simulink model "sistema2"  (R2026a)
settings: Solver=VariableStepAuto  StopTime=10
libraries: simulink x1, slpidlib x1

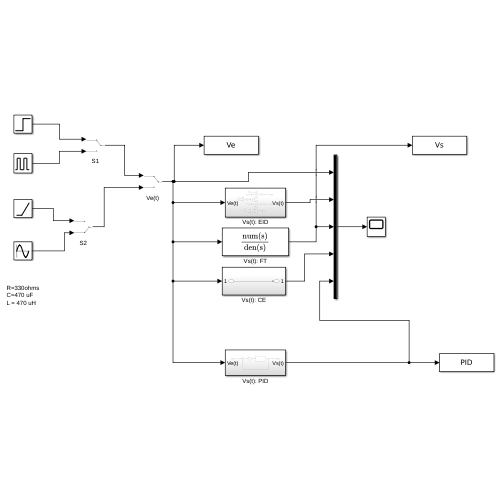
[thumbnail: Simulink's stored preview of the top-level diagram]
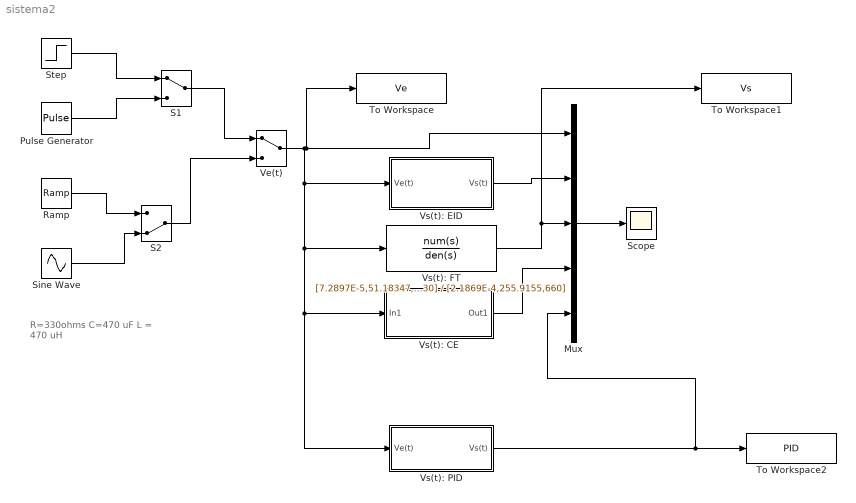
== system sistema2 ==
  note: R=330ohms
      | C=470 uF
      | L = 470 uH
  Mux : Mux  Inputs=5
  Pulse Generator : DiscretePulseGenerator  PulseType=Time based  Period=10  PulseWidth=10  PhaseDelay=1
  Ramp : simulink/Sources/Ramp  slope=1/10  start=0  InitialOutput=0
  S1 : ManualSwitch
  S2 : ManualSwitch  CurrentSetting=0
  Scope : Scope
      settings: ActiveDisplayYMinimum=-1.104134739416077  ActiveDisplayYMaximum=2.0672934495653212
  Sine Wave : Sin  Frequency=pi/2  SampleTime=0
  Step : Step  Time=0  SampleTime=0
  To Workspace : ToWorkspace  VariableName=Ve  SampleTime=-1
  To Workspace1 : ToWorkspace  VariableName=Vs  SampleTime=-1
  To Workspace2 : ToWorkspace  VariableName=PID  SampleTime=-1
  Ve(t) : ManualSwitch
  Vs(t): CE : Subsystem
  Vs(t): EID : Subsystem
  Vs(t): FT : TransferFcn  Numerator=[7.2897E-5,51.18347,330]  Denominator=[2.1869E-4,255.9155,660]
  Vs(t): PID : Subsystem
  wires:
  Vs(t): PID/1(Vs(t)) -> To Workspace2/1, Mux/5
  Mux/1 -> Scope/1
  S2/1 -> Ve(t)/2
  Ramp/1 -> S2/1
  Pulse Generator/1 -> S1/2
  Vs(t): CE/1(Out1) -> Mux/4
  Step/1 -> S1/1
  Vs(t): FT/1 -> To Workspace1/1, Mux/3
  S1/1 -> Ve(t)/1
  Vs(t): EID/1(Vs(t)) -> Mux/2
  Sine Wave/1 -> S2/2
  Ve(t)/1 -> Vs(t): EID/1(Ve(t)), Vs(t): FT/1, Vs(t): PID/1(Ve(t)), Vs(t): CE/1(In1), To Workspace/1, Mux/1

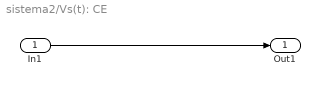
== system sistema2/Vs(t): CE ==
  In1 : Inport
  Out1 : Outport
  wires:
  In1/1 -> Out1/1

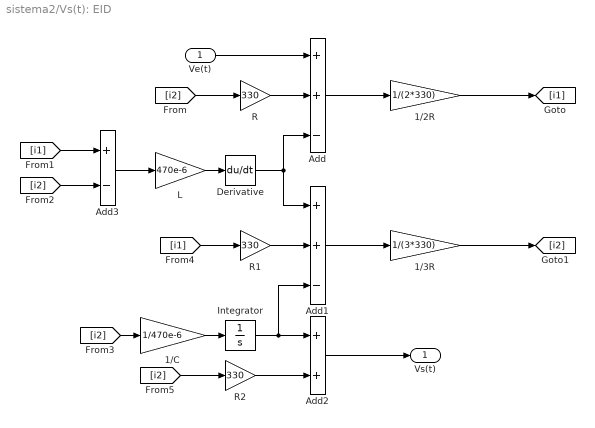
== system sistema2/Vs(t): EID ==
  Ve(t) : Inport
  1/2R : Gain  Gain=1/(2*330)
  1/3R : Gain  Gain=1/(3*330)
  1/C : Gain  Gain=1/470e-6
  Add : Sum  Inputs=++-
  Add1 : Sum  Inputs=++-
  Add2 : Sum
  Add3 : Sum  Inputs=+-
  Derivative : Derivative
  Integrator : Integrator
  L : Gain  Gain=470e-6
  R : Gain  Gain=330
  R1 : Gain  Gain=330
  R2 : Gain  Gain=330
  Vs(t) : Outport
  wires:
  Ve(t)/1 -> Add/1
  Add1/1 -> 1/3R/1
  1/3R/1 -> [i2]
  Add/1 -> 1/2R/1
  1/2R/1 -> [i1]
  R/1 -> Add/2
  [i2] -> R/1
  Derivative/1 -> Add1/1, Add/3
  R1/1 -> Add1/2
  Add3/1 -> L/1
  L/1 -> Derivative/1
  [i2] -> Add3/2
  [i1] -> Add3/1
  Integrator/1 -> Add1/3, Add2/1
  [i2] -> 1/C/1
  1/C/1 -> Integrator/1
  [i1] -> R1/1
  [i2] -> R2/1
  R2/1 -> Add2/2
  Add2/1 -> Vs(t)/1

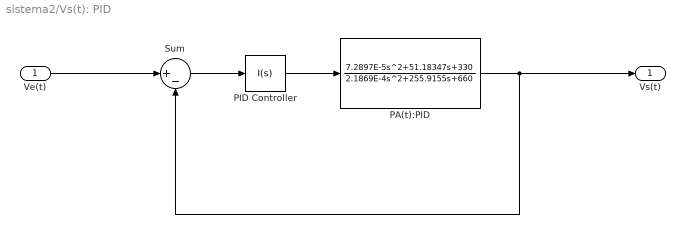
== system sistema2/Vs(t): PID ==
  Ve(t) : Inport
  PA(t):PID : TransferFcn  Numerator=[7.2897E-5,51.18347,330]  Denominator=[2.1869E-4,255.9155,660]
  PID Controller : slpidlib/PID Controller  Controller=I  Form=Parallel  TimeDomain=Continuous-time  UseExternalTs=off  SampleTime=-1  IntegratorMethod=Forward Euler  FilterMethod=Forward Euler  ControllerParametersSource=internal  P=289.6613  I=608.5886  UseKiTs=off  D=0.39134  UseExternalDerivativeSource=off  N=502.9743  UseFilter=on  TunerSelectOption=Transfer Function Based (PID Tuner App)  InitialConditionSource=internal  InitialConditionForIntegrator=0  InitialConditionForFilter=0  DifferentiatorICPrevScaledInput=0  ExternalReset=none  TrackingMode=off  Kt=1  LimitOutput=off  SatLimitsSource=internal  UpperSaturationLimit=inf  LowerSaturationLimit=-inf  LinearizeAsGain=on  AntiWindupMode=none  Kb=1  LimitIntegrator=off  UpperIntegratorSaturationLimit=inf  LowerIntegratorSaturationLimit=-inf  POutMin=[]  POutMax=[]  IOutMin=[]  IOutMax=[]  DOutMin=[]  DOutMax=[]  NOutMin=[]  NOutMax=[]  SumOutMin=[]  SumOutMax=[]  SaturationOutMin=[]  SaturationOutMax=[]  PParamMin=[]  PParamMax=[]  IParamMin=[]  IParamMax=[]  DParamMin=[]  DParamMax=[]  NParamMin=[]  NParamMax=[]  KbParamMin=[]  KbParamMax=[]  KtParamMin=[]  KtParamMax=[]  KbOutMin=[]  KbOutMax=[]  KtOutMin=[]  KtOutMax=[]  IntegratorOutMin=[]  IntegratorOutMax=[]  FilterOutMin=[]  FilterOutMax=[]  SumI1OutMin=[]  SumI1OutMax=[]  SumI2OutMin=[]  SumI2OutMax=[]  SumI3OutMin=[]  SumI3OutMax=[]  SumI4OutMin=[]  SumI4OutMax=[]  SumDOutMin=[]  SumDOutMax=[]  DifferentiatorOutMin=[]  DifferentiatorOutMax=[]  FilterDiffOutCoefMin=[]  FilterDiffOutCoefMax=[]  ReciprocalOutMin=[]  ReciprocalOutMax=[]  SumDenOutMin=[]  SumDenOutMax=[]  SumNumOutMin=[]  SumNumOutMax=[]  DivideOutMin=[]  DivideOutMax=[]  UdiffTsProdOutMin=[]  UdiffTsProdOutMax=[]  NTsProdOutMin=[]  NTsProdOutMax=[]  UintegralTsProdOutMin=[]  UintegralTsProdOutMax=[]  UngainTsProdOutMin=[]  UngainTsProdOutMax=[]  ClampingZeroOutDataTypeStr=Inherit: Inherit via back propagation  ClampingZeroOutMin=[]  ClampingZeroOutMax=[]  FilterDenConstantOutDataTypeStr=Inherit: Inherit via back propagation  FilterDenConstantOutMin=[]  FilterDenConstantOutMax=[]  PCopyOutDataTypeStr=Inherit: Inherit via back propagation  PCopyOutMin=[]  PCopyOutMax=[]  NCopyOutDataTypeStr=Inherit: Inherit via back propagation  NCopyOutMin=[]  NCopyOutMax=[]  IntegratorContinuousStateAttributes=''  IntegratorStateMustResolveToSignalObject=off  IntegratorRTWStateStorageClass=Auto  FilterContinuousStateAttributes=''  FilterStateMustResolveToSignalObject=off  FilterRTWStateStorageClass=Auto  ParallelPVariant=Disabled  IdealPVariant=Disabled  IVariant=InternalParameters  DVariant=Disabled  IntegratorVariant=Continuous  SatVariant=Disabled  AWVariant=Passthrough  PCopyVariant=Disabled  TRVariant=Disabled  FdbkBlocksVariant=Forward  IdealPFdbkVariant=Disabled  SatFdbkVariant=Disabled  DerivativeFilterVariant=Disabled  NVariant=Disabled  NCopyVariant=Disabled_SignalSpec  FilterICVariant=Disabled  IntegratorICVariant=InternalICs  ExternalResetVariant=Disabled  TRSumVariant=Passthrough  SumFdbkVariant=Disabled  SumVariant=Passthrough_I  TsampFilterVariant=InternalTs  TsampNgainVariant=Passthrough  TsampIntegralVariant=Disabled_SignalSpec  ExternalSaturationOutDataTypeStr=Inherit: Same as second input  DerivativeSourceVariant=Disabled  PreIntVariant=InternalPreInt
  Sum : Sum  Inputs=|+-
  Vs(t) : Outport
  wires:
  PA(t):PID/1 -> Vs(t)/1, Sum/2
  Sum/1 -> PID Controller/1
  PID Controller/1 -> PA(t):PID/1
  Ve(t)/1 -> Sum/1
